simulink model "simple"  (R2019a)
settings: Solver=VariableStepAuto  StartTime=0.0  StopTime=100  RelTol=1e-3  EnableMultiTasking=on
undefined symbols (not defined in the file or in its folder): m, n
libraries: simulink x2
settings Model: Creator=The MathWorks, Inc.  LastModifiedBy=Mojzar
settings DataIOCC: LimitDataPoints=on  SaveFormat=Array  ReturnWorkspaceOutputs=off
settings OptimizationCC: LifeSpan=inf
settings DebuggingCC: AllowSymbolicDim=off  SFUnexpectedBacktrackingDiag=warning  SFNoUnconditionalDefaultTransitionDiag=warning  SFExecutionAtInitializationDiag=none  ArithmeticOperatorsInVariantConditions=warning
settings ModelReferenceCC: PropagateSignalLabelsOutOfModel=off
settings SFSimCC: SimUseLocalCustomCode=off
settings RTWCC: RTWUseLocalCustomCode=off
settings CodeAppCC: StateflowObjectComments=on
settings GRTTargetCC: TargetLangStandard=C89/C90 (ANSI)  GeneratePreprocessorConditionals=Disable all
settings ConfigComp: CovMetricSettings=dw  CovHtmlReporting=on  CovSaveCumulativeToWorkspaceVar=on  CovSaveSingleToWorkspaceVar=on  CovExternalEMLEnable=off  CovSFcnEnable=off

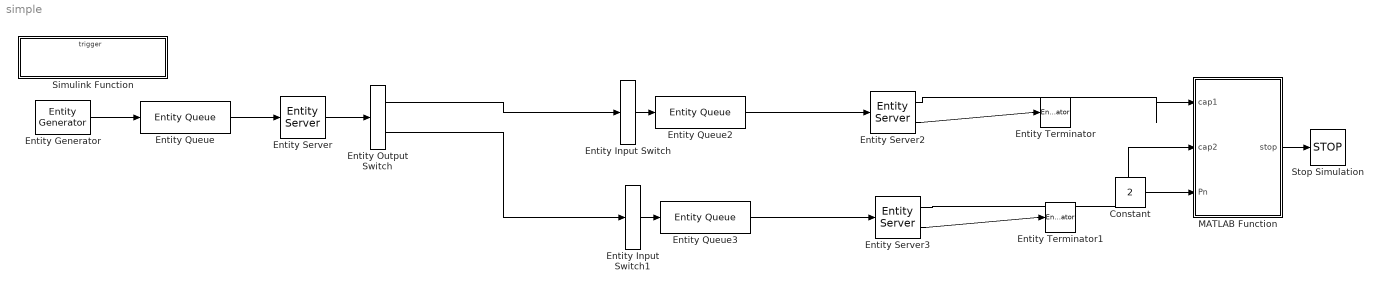
== system simple ==
  Constant : Constant  Value=2  SampleTime=-1
  Entity Input Switch : EntityInputSwitch  InputPortMessageModes=m  OutputPortMessageModes=m  NumberInputPorts=1
      settings: InputPortMap=u1
  Entity Input Switch1 : EntityInputSwitch  InputPortMessageModes=m  OutputPortMessageModes=m  NumberInputPorts=1
      settings: InputPortMap=u1
  Entity Output Switch : EntityOutputSwitch  InputPortMessageModes=m  OutputPortMessageModes=m,m  SwitchingCriterion=Round robin  SwitchAttributeName=Attribute1
  Entity Generator : EntityGenerator  OutputPortMessageModes=m  TimeSource=MATLAB action  IntergenerationTimeAction=dt = exponentialArrivalTime();  EntityType=Structured  EntityTypeName=Entity
  Entity Queue : EntityQueue  InputPortMessageModes=m  OutputPortMessageModes=m  Capacity=Inf  MulticastTag=B
      settings: OutputPortMap=o5
  Entity Queue2 : EntityQueue  InputPortMessageModes=m  OutputPortMessageModes=m  Capacity=2  MulticastTag=B
      settings: OutputPortMap=o5
  Entity Queue3 : EntityQueue  InputPortMessageModes=m  OutputPortMessageModes=m  Capacity=2  MulticastTag=B
      settings: OutputPortMap=o5
  Entity Server : EntityServer  InputPortMessageModes=m  OutputPortMessageModes=m  Capacity=3  ServiceTimeSource=MATLAB action  ServiceTimeAction=|
      | % Exponential service time with rate 1
      | mean = 1;
      | dt   = -mean * log(1 - rand());
  Entity Server2 : EntityServer  InputPortMessageModes=m  OutputPortMessageModes=n,m  Capacity=3  ServiceTimeSource=MATLAB action  ServiceTimeAction=|  NumberEntitiesInBlock=on
      | % Exponential service time with rate 1
      | mean = 0.2;
      | dt   = -mean * log(1 - rand());
      settings: OutputPortMap=o1,o9
  Entity Server3 : EntityServer  InputPortMessageModes=m  OutputPortMessageModes=n,m  Capacity=2  ServiceTimeSource=MATLAB action  ServiceTimeAction=|  NumberEntitiesInBlock=on
      | % Exponential service time with rate 1
      | mean = 0.1;
      | dt   = -mean * log(1 - rand());
      settings: OutputPortMap=o1,o9
  Entity Terminator : EntityTerminator  InputPortMessageModes=m
  Entity Terminator1 : EntityTerminator  InputPortMessageModes=m
  MATLAB Function : MATLAB Function  TreatAsAtomicUnit=on
  Simulink Function : Subsystem  TreatAsAtomicUnit=on
  Stop Simulation : Stop
  wires:
  Entity Queue/1 -> Entity Server/1
  Entity Generator/1 -> Entity Queue/1
  Entity Server/1 -> Entity Output Switch/1
  Entity Queue2/1 -> Entity Server2/1
  Entity Server2/2 -> Entity Terminator/1
  Entity Queue3/1 -> Entity Server3/1
  Entity Server3/2 -> Entity Terminator1/1
  Entity Input Switch/1 -> Entity Queue2/1
  Entity Input Switch1/1 -> Entity Queue3/1
  Entity Output Switch/1 -> Entity Input Switch/1
  Entity Output Switch/2 -> Entity Input Switch1/1
  Constant/1 -> MATLAB Function/3(Pn)
  MATLAB Function/1(stop) -> Stop Simulation/1
  Entity Server2/1 -> MATLAB Function/1(cap1)
  Entity Server3/1 -> MATLAB Function/2(cap2)

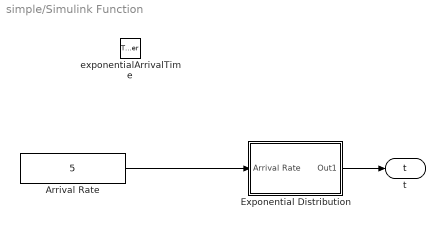
== system simple/Simulink Function ==
  exponentialArrivalTime : TriggerPort  TriggerType=function-call  IsSimulinkFunction=on  FunctionName=exponentialArrivalTime  VariantControl=Variant
  Arrival Rate : Constant  Value=5  SampleTime=-1
  Exponential Distribution : Subsystem
  t : ArgOut  DisableCoverage=on  ArgumentName=t
  wires:
  Arrival Rate/1 -> Exponential Distribution/1(Arrival Rate)
  Exponential Distribution/1(Out1) -> t/1

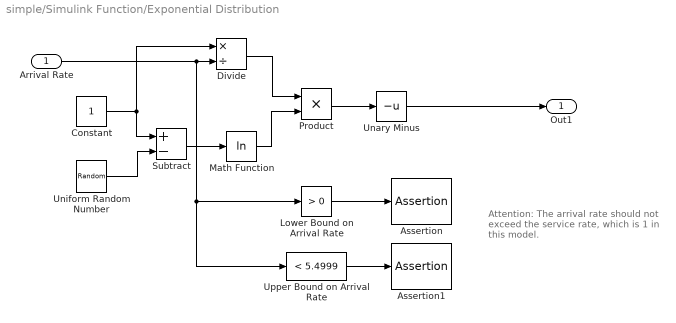
== system simple/Simulink Function/Exponential Distribution ==
  note: Attention: The arrival rate
      | should not exceed the service
      | rate, which is 1 in this model.
  Arrival Rate : Inport
  Assertion : Assertion
  Assertion1 : Assertion
  Constant : Constant
  Divide : Product  Inputs=*/
  Lower Bound on Arrival Rate : simulink/Logic and Bit Operations/Compare To Constant  relop=>  const=0  OutDataTypeStr=uint8  ZeroCross=off
  Math Function : Math  Operator=log  SaturateOnIntegerOverflow=on
  Product : Product  RndMeth=Zero
  Subtract : Sum  Inputs=+-
  Unary Minus : UnaryMinus
  Uniform Random Number : UniformRandomNumber  Minimum=0  Seed=randi(5000)
  "Upper Bound on Arrival Rate " : simulink/Logic and Bit Operations/Compare To Constant  relop=<  const=5.4999  OutDataTypeStr=uint8  ZeroCross=off
  Out1 : Outport
  wires:
  Arrival Rate/1 -> Divide/2, Lower Bound on Arrival Rate/1, "Upper Bound on Arrival Rate "/1
  Unary Minus/1 -> Out1/1
  Product/1 -> Unary Minus/1
  Math Function/1 -> Product/2
  Divide/1 -> Product/1
  Constant/1 -> Divide/1, Subtract/1
  Uniform Random Number/1 -> Subtract/2
  Lower Bound on Arrival Rate/1 -> Assertion/1
  "Upper Bound on Arrival Rate "/1 -> Assertion1/1
  Subtract/1 -> Math Function/1

== matlab function simple/MATLAB Function ==
  data: cap1 input; stop output; cap2 input; Pn input
function stop  = fcn(cap1,cap2,Pn)
max1 = 3;
max2= 2;
stop = 0;
if Pn == 1
    if cap1 == max1
        stop = 1;
    end
end
if Pn == 2
    if cap2 == max2
        stop = 1;
    end
end


end
